simulink model "EV_TMS_MODEL"  (R2024a)
settings: Solver=VariableStepAuto  StartTime=0.0  StopTime=1000  RelTol=1e-3
values from neighbouring files (symbols this model uses):
  air_density = 1.225    [model_script.m]
  battery_C1_LUT = [1913.6 12447 30609 ... (first row only)    [model_script.m]
  battery_capacity_LUT = [280.081 276.25 276.392]    [model_script.m]
  battery_cell_cp = 795    [model_script.m]
  battery_cell_mass = 2.5    [model_script.m]
  battery_Em_LUT = [3.4966 3.5057 3.5148 ... (first row only)    [model_script.m]
  battery_N_cells = 20    [model_script.m]
  battery_Qe_init = 0    [model_script.m]
  battery_R0_LUT = [0.0117 0.0085 0.009 ... (first row only)    [model_script.m]
  battery_R1_LUT = [0.0109 0.0029 0.0013 ... (first row only)    [model_script.m]
  battery_SOC_LUT = [0; 0.1; 0.25; 0.5; 0.75; 0.9; 1]    [model_script.m]
  battery_T_init = -10    [model_script.m]
  battery_temperature_LUT = [-10 0 5 20 40]    [model_script.m]
  cabin_doors_conductivity = 0.2    [model_script.m]
  cabin_glass_conductivity = 1    [model_script.m]
  cabin_roof_conductivity = 0.2    [model_script.m]
  cabin_T_init = -10    [model_script.m]
  coolant_channel_D = 0.0092    [model_script.m]
  coolant_pipe_D = 0.02    [model_script.m]
  coolant_T_init = 30    [model_script.m]
  coolant_tank_volume = 5    [model_script.m]
  CoolingPower_kW = 3    [model_script.m]
  duct_W = 0.2    [model_script.m]
  evap_superheat_temp = 5    [model_script.m]
  pump_speed_max = 3000    [model_script.m]
  refrigerant_massflowrate = CoolingPower_kW/(evap_outlet_enthalpy-evap_inlet_enthalpy)    (= 0.0184049079755)    [model_script.m]
  RPM_Compressor_nominal = 1000    [model_script.m]
  RPM_CondFan = 3000    [model_script.m]
  RPM_EvapFan = 3000    [model_script.m]
  T_set = 20    [model_script.m]
  tube_D = 0.01    [model_script.m]
  VolFlowrate_CondenserFan = condenser_air_massflowrate/air_density    (= 0.408163265306)    [model_script.m]
  VolFlowRate_CoolantRadiatorFan = 0.5    [model_script.m]
  VolFlowRate_EvapFan = evap_air_massflowrate/air_density    (= 0.487359122754)    [model_script.m]
undefined symbols (not defined in the file or in its folder): bulb, inlet
libraries: fl_lib x238, nesl_utility x75, SimscapeFluids_lib x25, LiBatteryElements_lib x16, simulink_extras x9, slpidlib x3, autolibshared x1, SignalEditorBlockLib x1
(part 1 of 7)
settings Model: Creator=sairathik  LastModifiedBy=sairathik
settings DataIOCC: LoggingToFile=on
settings SimscapeCC: SimscapeLogType=all

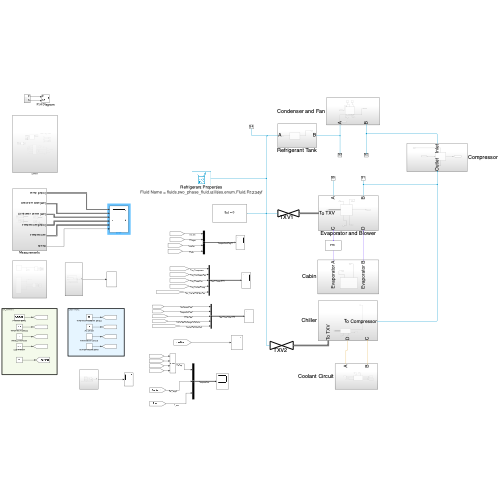
[thumbnail: Simulink's stored preview of the top-level diagram]
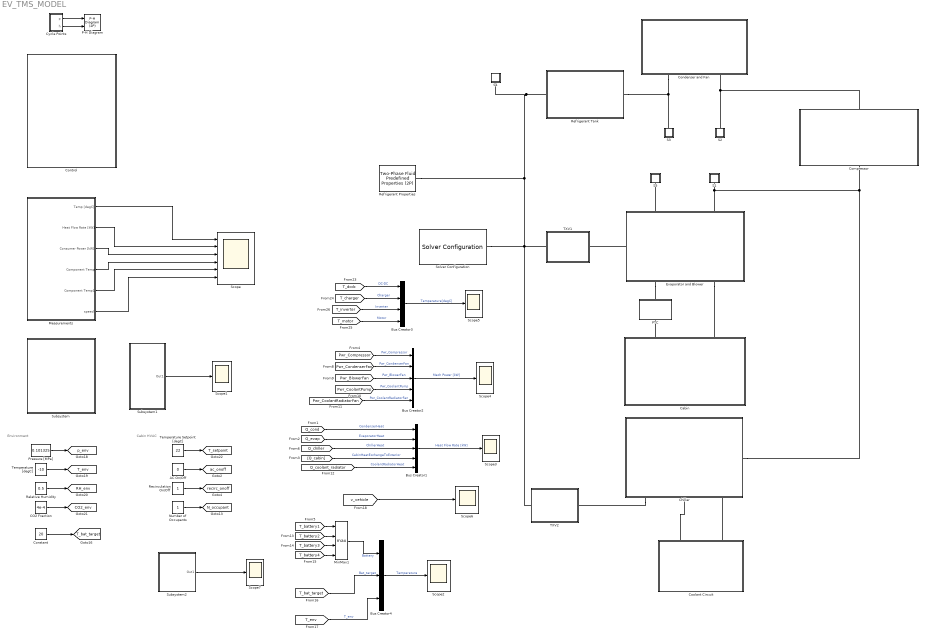
== system EV_TMS_MODEL ==
  note: Cabin HVAC
  note: Environment
  AC On/Off : Constant  Value=0
  Bus Creator1 : BusCreator  Inputs=5
  Bus Creator2 : BusCreator  Inputs=5
  Bus Creator3 : BusCreator  Inputs=4
  Bus Creator4 : BusCreator  Inputs=3
  CO2 Fraction : Constant  Value=4e-4
  Cabin : Subsystem
  Chiller : Subsystem
      settings: PortSchema="{\"entries\":[{\"content\":{\"sides\":[{\"content\":{\"connectorIds\":[\"LConn1\",\"LConn2\",\"LConn3\"]},\"type\":\"ConnectorPlacement.EquallySpacedRectSide\",\"uuid\":\"34bef901-d7f5-4aae-8cd5-5259b1e8621f\"},{\"content\":{\"side\":\"RIGHT\"},\"type\":\"ConnectorPlacement.EquallySpacedRectSide\",\"uuid\":\"b01a48cc-07de-4dff-b61c-731d99d876f5\"},{\"content\":{\"side\":\"TOP\"},\"type\":\"ConnectorPlacement.EquallySpacedRectSide\",\"uuid\":\"208c4f13-23a8-48df-b330-7ce2967b477c\"},{\"content\":{\"connectorIds\":[\"RConn1\"],\"side\":\"BOTTOM\"},\"type\":\"ConnectorPlacement.EquallySpacedRectSide\",\"uuid\":\"3f2d2c72-c43a-4e73-a9fe-b270fdc2a992\"}]},\"type\":\"ConnectorPlacement.EquallySpacedConnector\",\"uuid\":\"b9cc5a63-1194-4be5-9345-4e1b905bf50a\"}],\"packageUris\":[\"http://schema.mathworks.com/mf0/Connector/R2020b\"],\"version\":\"1.0\"}"
  Compressor : Subsystem
  Condenser and Fan : Subsystem
  Constant : Constant  Value=20
  Control : Subsystem
  Coolant Circuit : Subsystem
  Cycle Points : Subsystem
  Evaporator and Blower : Subsystem
      settings: PortSchema="{\"entries\":[{\"content\":{\"sides\":[{\"content\":{\"connectorIds\":[\"LConn1\"]},\"type\":\"ConnectorPlacement.EquallySpacedRectSide\",\"uuid\":\"157f3fa2-0ecb-424c-8810-23d73986b741\"},{\"content\":{\"side\":\"RIGHT\"},\"type\":\"ConnectorPlacement.EquallySpacedRectSide\",\"uuid\":\"a4531bf6-8393-4021-8b08-3c66bf47a331\"},{\"content\":{\"connectorIds\":[\"LConn2\",\"LConn3\"],\"side\":\"TOP\"},\"type\":\"ConnectorPlacement.EquallySpacedRectSide\",\"uuid\":\"3b910221-5f3a-43b2-b1cc-6f755753cce0\"},{\"content\":{\"connectorIds\":[\"RConn1\",\"RConn2\"],\"side\":\"BOTTOM\"},\"type\":\"ConnectorPlacement.EquallySpacedRectSide\",\"uuid\":\"a4f12d0e-e514-4dfe-871d-1a4bb02b790e\"}]},\"type\":\"ConnectorPlacement.EquallySpacedConnector\",\"uuid\":\"e79167fd-0289-46ca-9807-ec7889629a3a\"}],\"packageUris\":[\"http://schema.mathworks.com/mf0/Connector/R2020b\"],\"version\":\"1.0\"}"
  Measurements : Subsystem
  MinMax1 : MinMax  Function=max  Inputs=4
  Number of Occupants : Constant
  P-H Diagram : SimscapeFluids_lib/Two-Phase Fluid/Utilities/P-H Diagram (2P)
  PTC : Subsystem  Tag=PublishSubsystem
      mask Display: disp(get_param(gcb, 'Name'))
  Pressure [MPa] : Constant  Value=0.101325
  Recirculation On/Off : Constant
  Refrigerant Properties : SimscapeFluids_lib/Two-Phase Fluid/Utilities/Two-Phase Fluid Predefined Properties (2P)  fluid=fluids.two_phase_fluid.utilities.enum.Fluid.R1234yf  p_atm=0.6102 MPa  properties_range_check=simscape.enum.assert.action.error  q_rev=0.01 Pa
      settings: AttributesFormatString=Fluid Name = %<fluid>
  Refrigerant Tank : Subsystem
  Relative Humidity : Constant  Value=0.5
  S1 : Subsystem
      mask Display: disp(get_param(gcb, 'Name'))
  S2 : Subsystem
      mask Display: disp(get_param(gcb, 'Name'))
  S3 : Subsystem
      settings: PortSchema="{\"entries\":[{\"content\":{\"sides\":[{\"content\":{\"connectorIds\":[]},\"type\":\"ConnectorPlacement.EquallySpacedRectSide\",\"uuid\":\"16f002de-4636-401c-8be6-20698decbc91\"},{\"content\":{\"connectorIds\":[],\"side\":\"RIGHT\"},\"type\":\"ConnectorPlacement.EquallySpacedRectSide\",\"uuid\":\"76477188-11a3-4efa-a92e-0d269d480ac3\"},{\"content\":{\"connectorIds\":[],\"side\":\"TOP\"},\"type\":\"ConnectorPlacement.EquallySpacedRectSide\",\"uuid\":\"05fe64e4-9858-4712-a671-6ec27cab8615\"},{\"content\":{\"connectorIds\":[\"RConn1\"],\"side\":\"BOTTOM\"},\"type\":\"ConnectorPlacement.EquallySpacedRectSide\",\"uuid\":\"ddad7bbe-c900-450c-9863-e8fdc2274286\"}]},\"type\":\"ConnectorPlacement.EquallySpacedConnector\",\"uuid\":\"12bdef6d-66b8-4c10-9167-065994fcb3b8\"}],\"packageUris\":[\"http://schema.mathworks.com/mf0/Connector/R2020b\"],\"version\":\"1.0\"}"
      mask Display: disp(get_param(gcb, 'Name'))
  S4 : Subsystem
      mask Display: disp(get_param(gcb, 'Name'))
  S5 : Subsystem
      mask Display: disp(get_param(gcb, 'Name'))
  Scope : Scope  NumInputPorts=6
  Scope{1..7} (7 alike) : Scope
  Solver Configuration : nesl_utility/Solver Configuration  PhysicalDomain=network_engine_domain  SubClassName=solver  LeftPortType=input  RightPortType=generic  Tones=[]  Harmonics=[]  SimulateNoise=off  Profile=off  UseLocalSampling=off  EnableSwitchedLinearOptims=on  FrequencyDomain=off  UseCCode=off  RelTol=0.001  AbsTol=0.001  MinStep=1e-09  ToWorkspace=off  RevertToSquareIcSolve=off  NumHomotopyIterations=100  PhasorMode=off  PhasorModeNumHarmonics=1  ConsistencySolver=NEWTON_XTOL_AFTER_FTOL  IndexReductionMethod=DerivativeReplacement  DoDC=off  ResidualTolerance=1e-6  ConsistencyTolSource=GLOBAL  ConsistencyAbsTol=0.001  ConsistencyRelTol=0.001  ConsistencyTolFactor=0.001  UseLocalSolver=off  LocalSolverChoice=NE_BACKWARD_EULER_ADVANCER  ResolveIndetEquations=on  FunctionEvalNumThread=1  LocalSolverSampleTime=0.01  DoFixedCost=off  MaxNonlinIter=100  MaxModeIter=10  ComputeImpulses=off  ImpulseIterations=2  LinearAlgebra=auto  LinearAlgebraNumThread=0  EquationFormulation=NE_TIME_EF  DelaysMemoryBudget=1024  AutomaticFiltering=on  FilteringTimeConstant=0.001  PartitionStorageMethod=AS_NEEDED  PartitionMemoryBudget=1024  PartitionMethod=ROBUST  MultibodyUseLocalSolver=off  MultibodyLocalSolverChoice=ODE1  MultibodyLocalSolverSampleTime=0.001
  Subsystem : Subsystem
  Subsystem1 : Subsystem
  Subsystem2 : Subsystem
  TXV1 : Subsystem  Tag=PublishSubsystem
      mask Display:
      | color('white')
      | plot(100, 100)
      | plot(-100, -100)
      | color('black')
      | 
      | plot([0 -100 -100 0], [0 50 -50 0])
      | plot([0 100 100 0], [0 50 -50 0])
      | 
      | text(-50,60,get_param(gcb, 'Name'))
  TXV2 : Subsystem  Tag=PublishSubsystem
      mask Display:
      | color('white')
      | plot(100, 100)
      | plot(-100, -100)
      | color('black')
      | 
      | plot([0 -100 -100 0], [0 50 -50 0])
      | plot([0 100 100 0], [0 50 -50 0])
      | 
      | text(-50,60,get_param(gcb, 'Name'))
  Temperature Setpoint [degC] : Constant  Value=22
  Temperature [degC] : Constant  Value=-10
  tag scope: CO2_env=global, N_occupant=global, RH_env=global, T_bat_target=global, T_env=global, T_setpoint=global, ac_onoff=global, p_env=global, recirc_onoff=global
  wires:
  Cycle Points/2(h) -> P-H Diagram/2
  Cycle Points/1(p) -> P-H Diagram/1
  AC On/Off/1 -> [ac_onoff]
  Pressure [MPa]/1 -> [p_env]
  CO2 Fraction/1 -> [CO2_env]
  Number of Occupants/1 -> [N_occupant]
  Relative Humidity/1 -> [RH_env]
  Temperature Setpoint [degC]/1 -> [T_setpoint]
  Recirculation On/Off/1 -> [recirc_onoff]
  Temperature [degC]/1 -> [T_env]
  Measurements/1(Temp [degC]) -> Scope/1
  Measurements/2(Heat Flow Rate [kW]) -> Scope/2
  Measurements/3(Consumer Power [kW]) -> Scope/3
  Measurements/4(Component Temp) -> Scope/4
  Constant/1 -> [T_bat_target]
  Measurements/5(Component Temp1) -> Scope/5
  Subsystem1/1(Out1) -> Scope1/1
  Bus Creator4/1 -> Scope2/1  "Temperature"
  MinMax1/1 -> Bus Creator4/1  "Battery"
  [T_battery1] -> MinMax1/1
  [T_battery3] -> MinMax1/3
  [T_battery2] -> MinMax1/2
  [T_env] -> Bus Creator4/3  "T_env"
  [T_bat_target] -> Bus Creator4/2  "Bat_target"
  [T_battery4] -> MinMax1/4
  [Q_cond] -> Bus Creator1/1  "CondenserHeat"
  [Q_evap] -> Bus Creator1/2  "EvaporatorHeat"
  [Q_chiller] -> Bus Creator1/3  "ChillerHeat"
  [Q_cabin] -> Bus Creator1/4  "CabinHeatExchangeToExterior"
  [Q_coolant_radiator] -> Bus Creator1/5  "CoolantRadiatorHeat"
  Bus Creator1/1 -> Scope3/1  "Heat Flow Rate [kW]"
  [Pwr_CoolantPump] -> Bus Creator2/4  "Pwr_CoolantPump"
  [Pwr_CoolantRadiatorFan] -> Bus Creator2/5  "Pwr_CoolantRadiatorFan"
  [Pwr_CondenserFan] -> Bus Creator2/2  "Pwr_CondenserFan"
  Bus Creator2/1 -> Scope4/1  "Mech Power [kW]"
  [Pwr_Compressor] -> Bus Creator2/1  "Pwr_Compressor"
  [Pwr_BlowerFan] -> Bus Creator2/3  "Pwr_BlowerFan"
  Bus Creator3/1 -> Scope5/1  "Temperature[degC]"
  [T_charger] -> Bus Creator3/2  "Charger"
  [T_dcdc] -> Bus Creator3/1  "DC-DC"
  [T_motor] -> Bus Creator3/4  "Motor"
  [T_inverter] -> Bus Creator3/3  "Inverter"
  Measurements/6(speed) -> Scope/6
  [v_vehicle] -> Scope6/1
  Subsystem2/1(Out1) -> Scope7/1
  connections:
  S1/LConn1 -- Chiller/RConn1 -- Compressor/LConn1 -- Evaporator and Blower/LConn3
  Solver Configuration/RConn1 -- TXV2/RConn1 -- Refrigerant Properties/RConn1 -- Refrigerant Tank/LConn1 -- S4/LConn1 -- TXV1/RConn1
  S2/LConn1 -- Compressor/RConn1 -- Condenser and Fan/RConn2
  Condenser and Fan/RConn1 -- Refrigerant Tank/RConn1 -- S3/RConn1
  S5/LConn1 -- Evaporator and Blower/LConn2
  Evaporator and Blower/LConn1 -- TXV1/LConn1
  Evaporator and Blower/RConn1 -- PTC/RConn1
  PTC/LConn1 -- Cabin/LConn1
  Evaporator and Blower/RConn2 -- Cabin/LConn2
  Chiller/LConn1 -- TXV2/LConn1
  Coolant Circuit/LConn1 -- Chiller/LConn2
  Coolant Circuit/LConn2 -- Chiller/LConn3

== system EV_TMS_MODEL/Cabin ==
  Cabin : Subsystem
      settings: PortSchema="{\"entries\":[{\"content\":{\"sides\":[{\"content\":{},\"type\":\"ConnectorPlacement.EquallySpacedRectSide\",\"uuid\":\"5cf57e4f-975f-4b0b-a8e8-bf86758a11fa\"},{\"content\":{\"side\":\"RIGHT\"},\"type\":\"ConnectorPlacement.EquallySpacedRectSide\",\"uuid\":\"7f477a27-3a34-4ed6-85c3-331630c97133\"},{\"content\":{\"connectorIds\":[\"LConn1\",\"LConn2\"],\"side\":\"TOP\"},\"type\":\"ConnectorPlacement.EquallySpacedRectSide\",\"uuid\":\"743b5c17-84cf-4a2e-818e-c1a69eb195e5\"}]},\"type\":\"ConnectorPlacement.EquallySpacedConnector\",\"uuid\":\"4a6d6dd0-79df-4460-8879-70a258476fa5\"}],\"packageUris\":[\"http://schema.mathworks.com/mf0/Connector/R2020b\"],\"version\":\"1.0\"}"
      mask Display: disp(get_param(gcb, 'Name'));
  Evaporator A : PMIOPort  Side=Left
  Evaporator B : PMIOPort  Port=2  Side=Left
  connections:
  Evaporator B/RConn1 -- Cabin/LConn2
  Evaporator A/RConn1 -- Cabin/LConn1

== system EV_TMS_MODEL/Chiller ==
  Chiller : Subsystem  Tag=PublishSubsystem
      settings: PortSchema="{\"entries\":[{\"content\":{\"sides\":[{\"content\":{\"connectorIds\":[\"Out1\",\"LConn1\"]},\"type\":\"ConnectorPlacement.EquallySpacedRectSide\",\"uuid\":\"684495fe-43ac-42d2-91f9-c1083f68d635\"},{\"content\":{\"connectorIds\":[\"RConn1\"],\"side\":\"RIGHT\"},\"type\":\"ConnectorPlacement.EquallySpacedRectSide\",\"uuid\":\"acb3d27a-41e1-4bfe-a4d6-36d5666e4ba3\"},{\"content\":{\"connectorIds\":[\"LConn2\",\"LConn3\"],\"side\":\"TOP\"},\"type\":\"ConnectorPlacement.EquallySpacedRectSide\",\"uuid\":\"cdadeb40-472c-4edb-91b8-a2216ea85c99\"},{\"content\":{\"side\":\"BOTTOM\"},\"type\":\"ConnectorPlacement.EquallySpacedRectSide\",\"uuid\":\"46a4312c-e637-44ea-bfb3-e887da9d9904\"}]},\"type\":\"ConnectorPlacement.EquallySpacedConnector\",\"uuid\":\"20e25167-e167-414a-8c66-12b35ae5ef5e\"}],\"packageUris\":[\"http://schema.mathworks.com/mf0/Connector/R2020b\"],\"version\":\"1.0\"}"
      mask Display: disp(get_param(gcb, 'Name'));
  To TXV : PMIOPort  Side=Left
  D : PMIOPort  Port=2  Side=Left
  C : PMIOPort  Port=3  Side=Left
  To Compressor : PMIOPort  Port=4  Side=Right
  tag scope: Q_chiller=global
  wires:
  Chiller/1(Heat flow rate [kW]) -> [Q_chiller]  "Q_chiller"
  connections:
  C/RConn1 -- Chiller/LConn2
  Chiller/LConn1 -- To Compressor/RConn1
  D/RConn1 -- Chiller/LConn3
  Chiller/RConn1 -- To TXV/RConn1

== system EV_TMS_MODEL/Compressor ==
  Compressor : Subsystem
      settings: PortSchema="{\"entries\":[{\"content\":{\"sides\":[{\"content\":{\"connectorIds\":[\"LConn1\"]},\"type\":\"ConnectorPlacement.EquallySpacedRectSide\",\"uuid\":\"87497da4-7fcd-4c39-9d14-dd80365934db\"},{\"content\":{\"connectorIds\":[\"RConn1\"],\"side\":\"RIGHT\"},\"type\":\"ConnectorPlacement.EquallySpacedRectSide\",\"uuid\":\"c29b3d2b-7130-4a2f-8dcb-58b301edb84d\"},{\"content\":{\"connectorIds\":[\"In1\"],\"side\":\"TOP\"},\"type\":\"ConnectorPlacement.EquallySpacedRectSide\",\"uuid\":\"6b0e1579-3829-4056-a1f0-26424a36bca1\"},{\"content\":{\"connectorIds\":[\"Out1\"],\"side\":\"BOTTOM\"},\"type\":\"ConnectorPlacement.EquallySpacedRectSide\",\"uuid\":\"6b49380d-e724-4e3a-86e0-6bc21724e354\"}]},\"type\":\"ConnectorPlacement.EquallySpacedConnector\",\"uuid\":\"16d6c8a7-8265-44ec-91d1-631bbb83e0af\"}],\"packageUris\":[\"http://schema.mathworks.com/mf0/Connector/R2020b\"],\"version\":\"1.0\"}"
      mask Display: disp(get_param(gcb, 'Name'));
  Inlet : PMIOPort  Side=Right
  Outlet : PMIOPort  Port=2  Side=Left
  tag scope: Pwr_Compressor=global
  wires:
  [compressor] -> Compressor/1(Compressor On/Off)
  Compressor/1(Power [kW]) -> [Pwr_Compressor]  "Pwr_Compressor"
  connections:
  Compressor/LConn1 -- Outlet/RConn1
  Compressor/RConn1 -- Inlet/RConn1

== system EV_TMS_MODEL/Condenser and Fan ==
  Air In : fl_lib/Moist Air/Elements/Reservoir (MA)  pressure_spec=foundation.enum.pressure_spec.specified  reservoir_pressure=0.101325 MPa  temperature_spec=foundation.enum.temperature_spec.specified  reservoir_temperature=T_env degC  moisture_spec=foundation.enum.moisture_spec.relative_humidity  reservoir_RH=0.5  reservoir_x_w=0.01  reservoir_y_w=0.01  reservoir_HR=0.01  reservoir_Tw=287 K  trace_gas_spec=foundation.enum.trace_gas_spec.mole_fraction  reservoir_x_g=0.001  reservoir_y_g=0  RH_ws=1  area_A=duct_W^2 m^2
      settings: AttributesFormatString=temperature= %<reservoir_temperature>
  Air Out : fl_lib/Moist Air/Elements/Reservoir (MA)  pressure_spec=foundation.enum.pressure_spec.specified  reservoir_pressure=0.101325 MPa  temperature_spec=foundation.enum.temperature_spec.specified  reservoir_temperature=T_env degC  moisture_spec=foundation.enum.moisture_spec.relative_humidity  reservoir_RH=0.5  reservoir_x_w=0.01  reservoir_y_w=0.01  reservoir_HR=0.01  reservoir_Tw=287 K  trace_gas_spec=foundation.enum.trace_gas_spec.mole_fraction  reservoir_x_g=0.001  reservoir_y_g=0  RH_ws=1  area_A=duct_W^2 m^2
      settings: AttributesFormatString=temperature= %<reservoir_temperature>
  Condenser and Fan : Subsystem
      mask Display: disp(get_param(gcb, 'Name'));
  A : PMIOPort  Side=Right
  B : PMIOPort  Port=2  Side=Right
  tag scope: Pwr_CondenserFan=global, Q_cond=global
  wires:
  Condenser and Fan/2(Fan Power [kW]) -> [Q_cond]  "Q_condenser"
  Condenser and Fan/1(Heat Power [kW]) -> [Pwr_CondenserFan]  "Pwr_CondenserFan"
  [condenser_fan] -> Condenser and Fan/1(Fan On/Off)
  connections:
  Air Out/LConn1 -- Condenser and Fan/LConn2
  Condenser and Fan/LConn1 -- Air In/LConn1
  B/RConn1 -- Condenser and Fan/RConn2
  A/RConn1 -- Condenser and Fan/RConn1

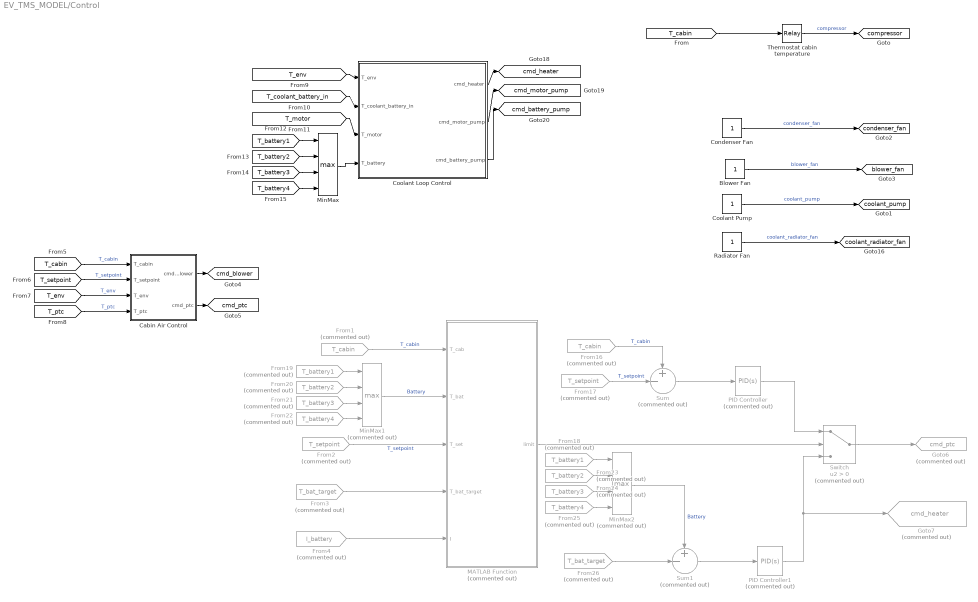
== system EV_TMS_MODEL/Control ==
  Blower Fan : Constant  SampleTime=1
  Cabin Air Control : Subsystem
  Condenser Fan : Constant  SampleTime=1
  Coolant Loop Control : Subsystem
  Coolant Pump : Constant  SampleTime=1
  From1 : From  Commented=on  GotoTag=T_cabin  TagVisibility=global
  From16 : From  Commented=on  GotoTag=T_cabin  TagVisibility=global
  From17 : From  Commented=on  GotoTag=T_setpoint  TagVisibility=global
  From18 : From  Commented=on  GotoTag=T_battery1  TagVisibility=global
  From19 : From  Commented=on  GotoTag=T_battery1  TagVisibility=global
  From2 : From  Commented=on  GotoTag=T_setpoint  TagVisibility=global
  From20 : From  Commented=on  GotoTag=T_battery2  TagVisibility=global
  From21 : From  Commented=on  GotoTag=T_battery3  TagVisibility=global
  From22 : From  Commented=on  GotoTag=T_battery4  TagVisibility=global
  From23 : From  Commented=on  GotoTag=T_battery2  TagVisibility=global
  From24 : From  Commented=on  GotoTag=T_battery3  TagVisibility=global
  From25 : From  Commented=on  GotoTag=T_battery4  TagVisibility=global
  From26 : From  Commented=on  GotoTag=T_bat_target  TagVisibility=global
  From3 : From  Commented=on  GotoTag=T_bat_target  TagVisibility=global
  From4 : From  Commented=on  GotoTag=I_battery  TagVisibility=global
  Goto6 : Goto  Commented=on  GotoTag=cmd_ptc  TagVisibility=global
  Goto7 : Goto  Commented=on  GotoTag=cmd_heater  TagVisibility=global
  MATLAB Function : MATLAB Function  Commented=on  TreatAsAtomicUnit=on
  MinMax : MinMax  Function=max  Inputs=4
  MinMax1 : MinMax  Commented=on  Function=max  Inputs=4
  MinMax2 : MinMax  Commented=on  Function=max  Inputs=4
  PID Controller : slpidlib/PID Controller  Commented=on  Controller=PID  Form=Parallel  TimeDomain=Continuous-time  UseExternalTs=off  SampleTime=-1  IntegratorMethod=Forward Euler  FilterMethod=Forward Euler  ControllerParametersSource=internal  P=1  I=1  UseKiTs=off  D=0  UseExternalDerivativeSource=off  N=100  UseFilter=on  TunerSelectOption=Transfer Function Based (PID Tuner App)  InitialConditionSource=internal  InitialConditionForIntegrator=0  InitialConditionForFilter=0  DifferentiatorICPrevScaledInput=0  ExternalReset=none  TrackingMode=off  Kt=1  LimitOutput=off  SatLimitsSource=internal  UpperSaturationLimit=inf  LowerSaturationLimit=-inf  LinearizeAsGain=on  AntiWindupMode=none  Kb=1  LimitIntegrator=off  UpperIntegratorSaturationLimit=inf  LowerIntegratorSaturationLimit=-inf  POutMin=[]  POutMax=[]  IOutMin=[]  IOutMax=[]  DOutMin=[]  DOutMax=[]  NOutMin=[]  NOutMax=[]  SumOutMin=[]  SumOutMax=[]  SaturationOutMin=[]  SaturationOutMax=[]  PParamMin=[]  PParamMax=[]  IParamMin=[]  IParamMax=[]  DParamMin=[]  DParamMax=[]  NParamMin=[]  NParamMax=[]  KbParamMin=[]  KbParamMax=[]  KtParamMin=[]  KtParamMax=[]  KbOutMin=[]  KbOutMax=[]  KtOutMin=[]  KtOutMax=[]  IntegratorOutMin=[]  IntegratorOutMax=[]  FilterOutMin=[]  FilterOutMax=[]  SumI1OutMin=[]  SumI1OutMax=[]  SumI2OutMin=[]  SumI2OutMax=[]  SumI3OutMin=[]  SumI3OutMax=[]  SumI4OutMin=[]  SumI4OutMax=[]  SumDOutMin=[]  SumDOutMax=[]  DifferentiatorOutMin=[]  DifferentiatorOutMax=[]  FilterDiffOutCoefMin=[]  FilterDiffOutCoefMax=[]  ReciprocalOutMin=[]  ReciprocalOutMax=[]  SumDenOutMin=[]  SumDenOutMax=[]  SumNumOutMin=[]  SumNumOutMax=[]  DivideOutMin=[]  DivideOutMax=[]  UdiffTsProdOutMin=[]  UdiffTsProdOutMax=[]  NTsProdOutMin=[]  NTsProdOutMax=[]  UintegralTsProdOutMin=[]  UintegralTsProdOutMax=[]  UngainTsProdOutMin=[]  UngainTsProdOutMax=[]  ClampingZeroOutDataTypeStr=Inherit: Inherit via back propagation  ClampingZeroOutMin=[]  ClampingZeroOutMax=[]  FilterDenConstantOutDataTypeStr=Inherit: Inherit via back propagation  FilterDenConstantOutMin=[]  FilterDenConstantOutMax=[]  PCopyOutDataTypeStr=Inherit: Inherit via back propagation  PCopyOutMin=[]  PCopyOutMax=[]  NCopyOutDataTypeStr=Inherit: Inherit via back propagation  NCopyOutMin=[]  NCopyOutMax=[]  IntegratorContinuousStateAttributes=''  IntegratorStateMustResolveToSignalObject=off  IntegratorRTWStateStorageClass=Auto  FilterContinuousStateAttributes=''  FilterStateMustResolveToSignalObject=off  FilterRTWStateStorageClass=Auto  ParallelPVariant=InternalParameters  IdealPVariant=Disabled  IVariant=InternalParameters  DVariant=InternalParameters  IntegratorVariant=Continuous  SatVariant=Disabled  AWVariant=Passthrough  PCopyVariant=Disabled  TRVariant=Disabled  FdbkBlocksVariant=Forward  IdealPFdbkVariant=Disabled  SatFdbkVariant=Disabled  DerivativeFilterVariant=ContFilter  NVariant=InternalParameters  NCopyVariant=Disabled  FilterICVariant=InternalICsFilter  IntegratorICVariant=InternalICs  ExternalResetVariant=Disabled  TRSumVariant=Passthrough  SumFdbkVariant=Disabled  SumVariant=Sum_PID  TsampFilterVariant=InternalTs  TsampNgainVariant=Passthrough  TsampIntegralVariant=Disabled_SignalSpec  ExternalSaturationOutDataTypeStr=Inherit: Same as second input  DerivativeSourceVariant=ErrorSignal
  PID Controller1 : slpidlib/PID Controller  Commented=on  Controller=PID  Form=Parallel  TimeDomain=Continuous-time  UseExternalTs=off  SampleTime=-1  IntegratorMethod=Forward Euler  FilterMethod=Forward Euler  ControllerParametersSource=internal  P=1  I=1  UseKiTs=off  D=0.1  UseExternalDerivativeSource=off  N=100  UseFilter=on  TunerSelectOption=Transfer Function Based (PID Tuner App)  InitialConditionSource=internal  InitialConditionForIntegrator=0  InitialConditionForFilter=0  DifferentiatorICPrevScaledInput=0  ExternalReset=none  TrackingMode=off  Kt=1  LimitOutput=off  SatLimitsSource=internal  UpperSaturationLimit=inf  LowerSaturationLimit=-inf  LinearizeAsGain=on  AntiWindupMode=none  Kb=1  LimitIntegrator=off  UpperIntegratorSaturationLimit=inf  LowerIntegratorSaturationLimit=-inf  POutMin=[]  POutMax=[]  IOutMin=[]  IOutMax=[]  DOutMin=[]  DOutMax=[]  NOutMin=[]  NOutMax=[]  SumOutMin=[]  SumOutMax=[]  SaturationOutMin=[]  SaturationOutMax=[]  PParamMin=[]  PParamMax=[]  IParamMin=[]  IParamMax=[]  DParamMin=[]  DParamMax=[]  NParamMin=[]  NParamMax=[]  KbParamMin=[]  KbParamMax=[]  KtParamMin=[]  KtParamMax=[]  KbOutMin=[]  KbOutMax=[]  KtOutMin=[]  KtOutMax=[]  IntegratorOutMin=[]  IntegratorOutMax=[]  FilterOutMin=[]  FilterOutMax=[]  SumI1OutMin=[]  SumI1OutMax=[]  SumI2OutMin=[]  SumI2OutMax=[]  SumI3OutMin=[]  SumI3OutMax=[]  SumI4OutMin=[]  SumI4OutMax=[]  SumDOutMin=[]  SumDOutMax=[]  DifferentiatorOutMin=[]  DifferentiatorOutMax=[]  FilterDiffOutCoefMin=[]  FilterDiffOutCoefMax=[]  ReciprocalOutMin=[]  ReciprocalOutMax=[]  SumDenOutMin=[]  SumDenOutMax=[]  SumNumOutMin=[]  SumNumOutMax=[]  DivideOutMin=[]  DivideOutMax=[]  UdiffTsProdOutMin=[]  UdiffTsProdOutMax=[]  NTsProdOutMin=[]  NTsProdOutMax=[]  UintegralTsProdOutMin=[]  UintegralTsProdOutMax=[]  UngainTsProdOutMin=[]  UngainTsProdOutMax=[]  ClampingZeroOutDataTypeStr=Inherit: Inherit via back propagation  ClampingZeroOutMin=[]  ClampingZeroOutMax=[]  FilterDenConstantOutDataTypeStr=Inherit: Inherit via back propagation  FilterDenConstantOutMin=[]  FilterDenConstantOutMax=[]  PCopyOutDataTypeStr=Inherit: Inherit via back propagation  PCopyOutMin=[]  PCopyOutMax=[]  NCopyOutDataTypeStr=Inherit: Inherit via back propagation  NCopyOutMin=[]  NCopyOutMax=[]  IntegratorContinuousStateAttributes=''  IntegratorStateMustResolveToSignalObject=off  IntegratorRTWStateStorageClass=Auto  FilterContinuousStateAttributes=''  FilterStateMustResolveToSignalObject=off  FilterRTWStateStorageClass=Auto  ParallelPVariant=InternalParameters  IdealPVariant=Disabled  IVariant=InternalParameters  DVariant=InternalParameters  IntegratorVariant=Continuous  SatVariant=Disabled  AWVariant=Passthrough  PCopyVariant=Disabled  TRVariant=Disabled  FdbkBlocksVariant=Forward  IdealPFdbkVariant=Disabled  SatFdbkVariant=Disabled  DerivativeFilterVariant=ContFilter  NVariant=InternalParameters  NCopyVariant=Disabled  FilterICVariant=InternalICsFilter  IntegratorICVariant=InternalICs  ExternalResetVariant=Disabled  TRSumVariant=Passthrough  SumFdbkVariant=Disabled  SumVariant=Sum_PID  TsampFilterVariant=InternalTs  TsampNgainVariant=Passthrough  TsampIntegralVariant=Disabled_SignalSpec  ExternalSaturationOutDataTypeStr=Inherit: Same as second input  DerivativeSourceVariant=ErrorSignal
  Radiator Fan : Constant  SampleTime=1
  Sum : Sum  Commented=on  Inputs=+-|
  Sum1 : Sum  Commented=on  Inputs=+-|
  Switch : Switch  Commented=on  Criteria=u2 > Threshold  SaturateOnIntegerOverflow=off  InputSameDT=off
  Thermostat cabin temperature : Relay  OnSwitchValue=T_set + 1  OffSwitchValue=T_set  ZeroCross=off
  tag scope: blower_fan=global, cmd_battery_pump=global, cmd_blower=global, cmd_heater=global, cmd_motor_pump=global, cmd_ptc=global, compressor=global, condenser_fan=global, coolant_pump=global, coolant_radiator_fan=global
  wires:
  Thermostat cabin temperature/1 -> [compressor]  "compressor"
  [T_coolant_battery_in] -> Coolant Loop Control/2(T_coolant_battery_in)
  Coolant Loop Control/3(cmd_battery_pump) -> [cmd_battery_pump]
  [T_battery1] -> MinMax/1
  [T_battery4] -> MinMax/4
  [T_env] -> Coolant Loop Control/1(T_env)
  [T_cabin] -> Thermostat cabin temperature/1
  Coolant Loop Control/2(cmd_motor_pump) -> [cmd_motor_pump]
  [T_motor] -> Coolant Loop Control/3(T_motor)
  Radiator Fan/1 -> [coolant_radiator_fan]  "coolant_radiator_fan"
  [T_battery3] -> MinMax/3
  Coolant Pump/1 -> [coolant_pump]  "coolant_pump"
  [T_battery2] -> MinMax/2
  MinMax/1 -> Coolant Loop Control/4(T_battery)
  Condenser Fan/1 -> [condenser_fan]  "condenser_fan"
  Coolant Loop Control/1(cmd_heater) -> [cmd_heater]
  [T_env] -> Cabin Air Control/3(T_env)  "T_env"
  [T_cabin] -> Cabin Air Control/1(T_cabin)  "T_cabin"
  [T_setpoint] -> Cabin Air Control/2(T_setpoint)  "T_setpoint"
  Cabin Air Control/2(cmd_ptc) -> [cmd_ptc]
  [T_ptc] -> Cabin Air Control/4(T_ptc)  "T_ptc"
  Cabin Air Control/1(cmd_blower) -> [cmd_blower]
  From1/1 -> MATLAB Function/1(T_cab)  "T_cabin"
  From22/1 -> MinMax1/4
  From21/1 -> MinMax1/3
  From19/1 -> MinMax1/1
  MinMax1/1 -> MATLAB Function/2(T_bat)  "Battery"
  From20/1 -> MinMax1/2
  From2/1 -> MATLAB Function/3(T_set)  "T_setpoint"
  From3/1 -> MATLAB Function/4(T_bat_target)
  PID Controller/1 -> Switch/1
  MATLAB Function/1(limit) -> Switch/2
  PID Controller1/1 -> Switch/3, Goto7/1
  From4/1 -> MATLAB Function/5(I)
  Switch/1 -> Goto6/1
  From16/1 -> Sum/1  "T_cabin"
  From17/1 -> Sum/2  "T_setpoint"
  MinMax2/1 -> Sum1/1  "Battery"
  From25/1 -> MinMax2/4
  From18/1 -> MinMax2/1
  From24/1 -> MinMax2/3
  From23/1 -> MinMax2/2
  From26/1 -> Sum1/2
  Sum/1 -> PID Controller/1
  Sum1/1 -> PID Controller1/1
  Blower Fan/1 -> [blower_fan]  "blower_fan"

== system EV_TMS_MODEL/Coolant Circuit ==
  Coolant Circuit : Subsystem
      settings: PortSchema="{\"entries\":[{\"content\":{\"sides\":[{\"content\":{\"connectorIds\":[\"In1\",\"In2\",\"In3\"]},\"type\":\"ConnectorPlacement.EquallySpacedRectSide\",\"uuid\":\"61b3bd2b-efba-48b8-bc1e-7d5fd1f93ea8\"},{\"content\":{\"connectorIds\":[\"Out1\",\"Out2\",\"Out3\",\"Out4\"],\"side\":\"RIGHT\"},\"type\":\"ConnectorPlacement.EquallySpacedRectSide\",\"uuid\":\"116770ca-4665-4fbe-8ef7-14ad65bf6363\"},{\"content\":{\"connectorIds\":[\"LConn1\",\"LConn2\"],\"side\":\"TOP\"},\"type\":\"ConnectorPlacement.EquallySpacedRectSide\",\"uuid\":\"8588f2a2-4124-40f5-9c68-b1b3344e047c\"}]},\"type\":\"ConnectorPlacement.EquallySpacedConnector\",\"uuid\":\"af351b75-e118-4ad1-8604-555a25a7fec0\"}],\"packageUris\":[\"http://schema.mathworks.com/mf0/Connector/R2020b\"],\"version\":\"1.0\"}"
      mask Display: disp(get_param(gcb, 'Name'));
  Heat flow rate to coolant [kW] : Constant  Value=0.5  SampleTime=1
  A : PMIOPort  Side=Left
  B : PMIOPort  Port=2  Side=Left
  tag scope: Pwr_CoolantPump=global, Pwr_CoolantRadiatorFan=global, Q_coolant_radiator=global, T_coolant=global
  wires:
  Heat flow rate to coolant [kW]/1 -> Coolant Circuit/1(Heat flow rate [kW])  "heat_flow_to_coolant_kW"
  Coolant Circuit/4(Radiator Heat Rate [kW]) -> [Q_coolant_radiator]  "Q_coolant_radiator"
  [coolant_pump] -> Coolant Circuit/2(Coolant Pump On/Off)
  Coolant Circuit/2(Pump Power [kW]) -> [Pwr_CoolantPump]  "Pwr_CoolantPump"
  Coolant Circuit/3(Radiator Fan Pwr [kW]) -> [Pwr_CoolantRadiatorFan]  "Pwr_CoolantRadiatorFan"
  [coolant_radiator_fan] -> Coolant Circuit/3(Radiator Fan On/Off)
  Coolant Circuit/1(Temperature [degC]) -> [T_coolant]  "T_coolant"
  connections:
  Coolant Circuit/LConn1 -- A/RConn1
  Coolant Circuit/LConn2 -- B/RConn1

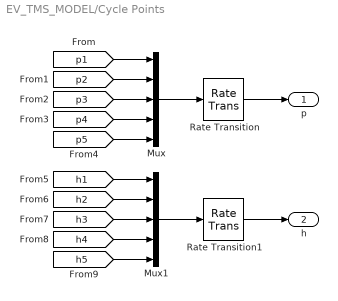
== system EV_TMS_MODEL/Cycle Points ==
  Mux : Mux  Inputs=5
  Mux1 : Mux  Inputs=5
  Rate Transition : RateTransition  OutPortSampleTime=10
  Rate Transition1 : RateTransition  OutPortSampleTime=10
  p : Outport
  h : Outport  Port=2
  wires:
  [p1] -> Mux/1
  [p2] -> Mux/2
  [p3] -> Mux/3
  [p4] -> Mux/4
  [p5] -> Mux/5
  Mux/1 -> Rate Transition/1
  Mux1/1 -> Rate Transition1/1
  [h5] -> Mux1/5
  [h4] -> Mux1/4
  [h3] -> Mux1/3
  [h2] -> Mux1/2
  [h1] -> Mux1/1
  Rate Transition/1 -> p/1
  Rate Transition1/1 -> h/1

== system EV_TMS_MODEL/Evaporator and Blower ==
  Evaporator and Blower Fan : Subsystem
      settings: PortSchema="{\"entries\":[{\"content\":{\"sides\":[{\"content\":{\"connectorIds\":[\"LConn1\",\"LConn2\"]},\"type\":\"ConnectorPlacement.EquallySpacedRectSide\",\"uuid\":\"94f743b0-016e-4f6c-ba37-cd5c9e5decb1\"},{\"content\":{\"connectorIds\":[\"RConn1\",\"RConn2\"],\"side\":\"RIGHT\"},\"type\":\"ConnectorPlacement.EquallySpacedRectSide\",\"uuid\":\"4e78d493-e8a5-489f-9c9b-6c9134237572\"},{\"content\":{\"connectorIds\":[\"LConn3\"],\"side\":\"TOP\"},\"type\":\"ConnectorPlacement.EquallySpacedRectSide\",\"uuid\":\"0b95dc75-9fe3-4b9e-8dc0-c99924a5b683\"},{\"content\":{\"connectorIds\":[\"Out1\"],\"side\":\"BOTTOM\"},\"type\":\"ConnectorPlacement.EquallySpacedRectSide\",\"uuid\":\"3125a7ac-4364-4843-9f9a-28cc842c280f\"}]},\"type\":\"ConnectorPlacement.EquallySpacedConnector\",\"uuid\":\"0b0f7158-6d74-402a-9204-25c9a3fd4099\"}],\"packageUris\":[\"http://schema.mathworks.com/mf0/Connector/R2020b\"],\"version\":\"1.0\"}"
      mask Display: disp(get_param(gcb, 'Name'));
  To TXV : PMIOPort  Side=Left
  A : PMIOPort  Port=2  Side=Left
  B : PMIOPort  Port=3  Side=Left
  C : PMIOPort  Port=4  Side=Right
  D : PMIOPort  Port=5  Side=Right
  tag scope: Q_evap=global
  wires:
  Evaporator and Blower Fan/1(Heat Power [kW]) -> [Q_evap]  "Q_evaporator"
  connections:
  B/RConn1 -- Evaporator and Blower Fan/LConn2
  Evaporator and Blower Fan/RConn1 -- C/RConn1
  Evaporator and Blower Fan/LConn3 -- To TXV/RConn1
  A/RConn1 -- Evaporator and Blower Fan/LConn1
  Evaporator and Blower Fan/RConn2 -- D/RConn1

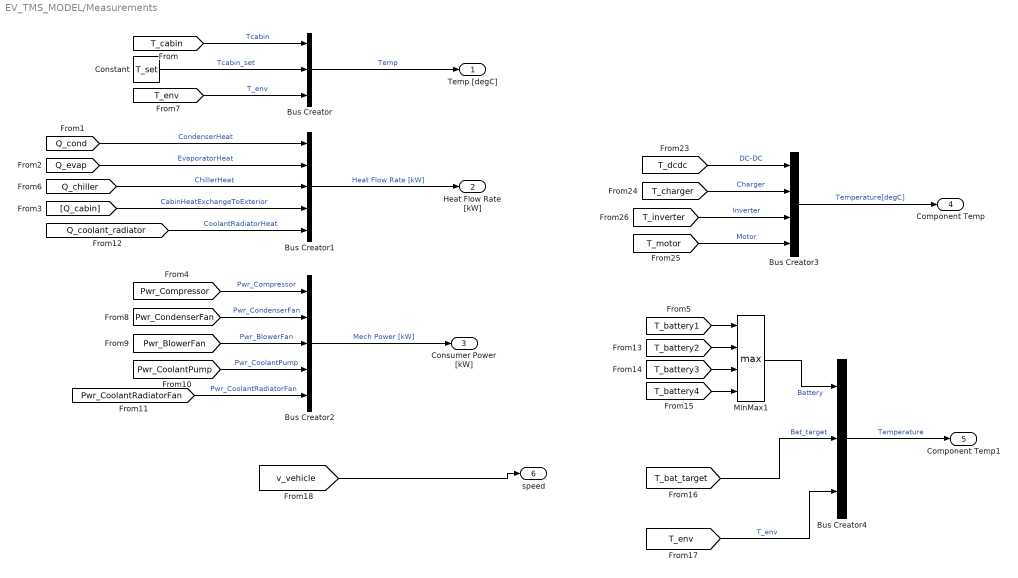
== system EV_TMS_MODEL/Measurements ==
  Bus Creator : BusCreator  Inputs=3
  Bus Creator1 : BusCreator  Inputs=5
  Bus Creator2 : BusCreator  Inputs=5
  Bus Creator3 : BusCreator  Inputs=4
  Bus Creator4 : BusCreator  Inputs=3
  Constant : Constant  Value=T_set
  MinMax1 : MinMax  Function=max  Inputs=4
  Temp [degC] : Outport
  Heat Flow Rate [kW] : Outport  Port=2
  Consumer Power [kW] : Outport  Port=3
  Component Temp : Outport  Port=4
  Component Temp1 : Outport  Port=5
  speed : Outport  Port=6
  wires:
  [T_cabin] -> Bus Creator/1  "Tcabin"
  Constant/1 -> Bus Creator/2  "Tcabin_set"
  Bus Creator/1 -> Temp [degC]/1  "Temp"
  Bus Creator1/1 -> Heat Flow Rate [kW]/1  "Heat Flow Rate [kW]"
  [Q_cond] -> Bus Creator1/1  "CondenserHeat"
  [Q_evap] -> Bus Creator1/2  "EvaporatorHeat"
  [Q_cabin] -> Bus Creator1/4  "CabinHeatExchangeToExterior"
  [Q_chiller] -> Bus Creator1/3  "ChillerHeat"
  [T_env] -> Bus Creator/3  "T_env"
  [Pwr_Compressor] -> Bus Creator2/1  "Pwr_Compressor"
  Bus Creator2/1 -> Consumer Power [kW]/1  "Mech Power [kW]"
  [Pwr_CondenserFan] -> Bus Creator2/2  "Pwr_CondenserFan"
  [Pwr_BlowerFan] -> Bus Creator2/3  "Pwr_BlowerFan"
  [Pwr_CoolantPump] -> Bus Creator2/4  "Pwr_CoolantPump"
  [Pwr_CoolantRadiatorFan] -> Bus Creator2/5  "Pwr_CoolantRadiatorFan"
  [Q_coolant_radiator] -> Bus Creator1/5  "CoolantRadiatorHeat"
  Bus Creator3/1 -> Component Temp/1  "Temperature[degC]"
  [T_dcdc] -> Bus Creator3/1  "DC-DC"
  [T_charger] -> Bus Creator3/2  "Charger"
  [T_motor] -> Bus Creator3/4  "Motor"
  [T_inverter] -> Bus Creator3/3  "Inverter"
  [T_battery4] -> MinMax1/4
  [T_battery3] -> MinMax1/3
  [T_battery1] -> MinMax1/1
  MinMax1/1 -> Bus Creator4/1  "Battery"
  [T_battery2] -> MinMax1/2
  [T_bat_target] -> Bus Creator4/2  "Bat_target"
  [T_env] -> Bus Creator4/3  "T_env"
  Bus Creator4/1 -> Component Temp1/1  "Temperature"
  [v_vehicle] -> speed/1

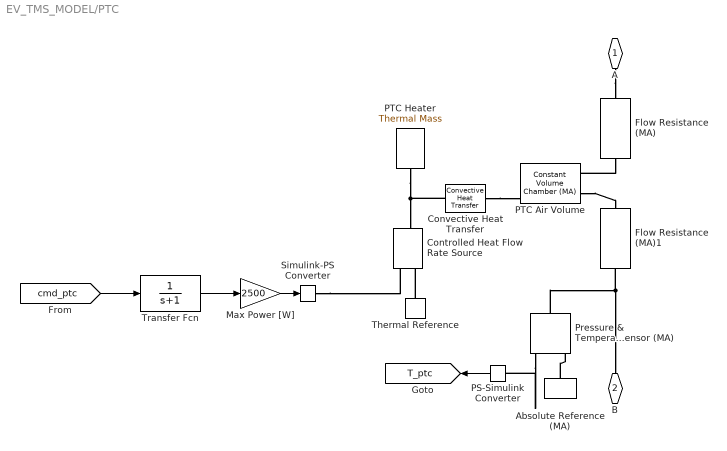
== system EV_TMS_MODEL/PTC ==
  Absolute Reference (MA) : fl_lib/Moist Air/Elements/Absolute Reference (MA)
  Controlled Heat Flow Rate Source : fl_lib/Thermal/Thermal Sources/Controlled Heat Flow Rate Source
  Convective Heat Transfer : fl_lib/Thermal/Thermal Elements/Convective Heat Transfer  thermal_type=foundation.enum.constant_variable.constant  area=1 m^2  heat_tr_coeff=200 W/(m^2 * K)  min_heat_tr_coeff=1e-3 W/(K*m^2)  T_specify=off  T_priority=None  T=0 K  T_nominal_specify=off  T_nominal_value=1  T_nominal_unit=K  Q_specify=off  Q_priority=None  Q=0 W  Q_nominal_specify=off  Q_nominal_value=1  Q_nominal_unit=W
  Flow Resistance (MA) : fl_lib/Moist Air/Elements/Flow Resistance (MA)  delta_p_nominal=2e-4 MPa  mdot_nominal=0.15 kg/s  rho_nominal=1.2 kg/m^3  area=cabin_duct_area m^2  laminar_fraction=1e-3
  Flow Resistance (MA)1 : fl_lib/Moist Air/Elements/Flow Resistance (MA)  delta_p_nominal=2e-4 MPa  mdot_nominal=0.15 kg/s  rho_nominal=1.2 kg/m^3  area=cabin_duct_area m^2  laminar_fraction=1e-3
  Max Power [W] : Gain  Gain=2500
  PS-Simulink Converter : nesl_utility/PS-Simulink Converter  PhysicalDomain=network_engine_domain  SubClassName=ps_output  LeftPortType=input  RightPortType=output  PseudoPeriodic=off  Frequencies=[]  VectorFormat=1-D array  Unit=degC  AffineConversion=on
  PTC Heater : fl_lib/Thermal/Thermal Elements/Thermal Mass  mass_type=foundation.enum.constant_variable.constant  mass=1.5 kg  sp_heat=447 J/kg/K  mass_min=1e-6 kg  num_ports=foundation.enum.numPorts2.one  m_specify=off  m_priority=High  m=1 kg  m_nominal_specify=off  m_nominal_value=1  m_nominal_unit=kg  T_specify=on  T_priority=High  T=cabin_T_init degC  T_nominal_specify=off  T_nominal_value=1  T_nominal_unit=K  Q_specify=off  Q_priority=None  Q=0 W  Q_nominal_specify=off  Q_nominal_value=1  Q_nominal_unit=W
  PTC Air Volume : fl_lib/Moist Air/Elements/Constant Volume Chamber (MA)  volume=0.001 m^3  num_ports=foundation.enum.num_ports.two  area_A=cabin_duct_area m^2  area_B=cabin_duct_area m^2  area_C=0.01 m^2  area_D=0.01 m^2  RH_ws=1  time_constant=1e-3 s  moisture_trace_gas_source=foundation.enum.moisture_trace_gas_source.none  moisture_source_spec=foundation.enum.moisture_source_spec.vapor  moisture_mass_flow=0 kg/s  moisture_temperature_spec=foundation.enum.temperature_spec.atmospheric  moisture_temperature=293.15 K  trace_gas_mass_flow=0 kg/s  trace_gas_temperature_spec=foundation.enum.temperature_spec.atmospheric  trace_gas_temperature=293.15 K  p_I_specify=on  p_I_priority=High  p_I=cabin_p_init MPa  p_I_nominal_specify=off  p_I_nominal_value=1  p_I_nominal_unit=MPa  T_I_specify=on  T_I_priority=High  T_I=cabin_T_init degC  T_I_nominal_specify=off  T_I_nominal_value=1  T_I_nominal_unit=K  RH_I_specify=on  RH_I_priority=High  RH_I=cabin_RH_init  RH_I_nominal_specify=off  RH_I_nominal_value=1  RH_I_nominal_unit=1  x_w_I_specify=off  x_w_I_priority=None  x_w_I=0  x_w_I_nominal_specify=off  x_w_I_nominal_value=1  x_w_I_nominal_unit=1  y_w_I_specify=off  y_w_I_priority=None  y_w_I=0  y_w_I_nominal_specify=off  y_w_I_nominal_value=1  y_w_I_nominal_unit=1  HR_I_specify=off  HR_I_priority=None  HR_I=0  HR_I_nominal_specify=off  HR_I_nominal_value=1  HR_I_nominal_unit=1  x_g_I_specify=on  x_g_I_priority=None  x_g_I=0  x_g_I_nominal_specify=off  x_g_I_nominal_value=1  x_g_I_nominal_unit=1  y_g_I_specify=on  y_g_I_priority=High  y_g_I=cabin_CO2_init  y_g_I_nominal_specify=off  y_g_I_nominal_value=1  y_g_I_nominal_unit=1
      settings: InternalSimscapePortConfiguration="{\"Bottom\":[],\"Left\":[{\"id\":\"A\",\"label\":\"A\",\"type\":\"foundation.moist_air.moist_air\"},{\"id\":\"B\",\"label\":\"B\",\"type\":\"foundation.moist_air.moist_air\"}],\"Right\":[{\"id\":\"W\",\"label\":\"W\",\"type\":\"output\"},{\"id\":\"F\",\"label\":\"F\",\"type\":\"output\"},{\"id\":\"H\",\"label\":\"H\",\"type\":\"foundation.thermal.thermal\"}],\"Top\":[]}"
  Pressure & Temperature Sensor (MA) : fl_lib/Moist Air/Sensors/Pressure & Temperature Sensor (MA)  reference=foundation.enum.MeasurementReference.difference  pressure=true  pressure_spec=foundation.enum.PressureMeasementSpec.Absolute  temperature=true
      settings: InternalSimscapePortConfiguration="{\"Bottom\":[{\"id\":\"T\",\"label\":\"T\",\"type\":\"output\"}],\"Left\":[{\"id\":\"A\",\"label\":\"A\",\"type\":\"foundation.moist_air.moist_air\"}],\"Right\":[{\"id\":\"B\",\"label\":\"B\",\"type\":\"foundation.moist_air.moist_air\"},{\"id\":\"P\",\"label\":\"P\",\"type\":\"output\"}],\"Top\":[]}"
  Simulink-PS Converter : nesl_utility/Simulink-PS Converter  PhysicalDomain=network_engine_domain  SubClassName=ps_input  LeftPortType=input  RightPortType=output  PseudoPeriodic=off  Frequencies=[]  NoiseDistribution=none  NoiseParameters=[]  Unit=W  AffineConversion=off  FilteringAndDerivatives=provide  SimscapeFilterOrder=1  InputFilterTimeConstant=0.001  UdotUserProvided=0
  Thermal Reference : fl_lib/Thermal/Thermal Elements/Thermal Reference
  Transfer Fcn : TransferFcn  Denominator=[1 1]
  A : PMIOPort  Side=Left
  B : PMIOPort  Port=2  Side=Right
  tag scope: T_ptc=global
  wires:
  Max Power [W]/1 -> Simulink-PS Converter/1
  Transfer Fcn/1 -> Max Power [W]/1
  [cmd_ptc] -> Transfer Fcn/1
  PS-Simulink Converter/1 -> [T_ptc]
  connections:
  PTC Heater/LConn1 -- Convective Heat Transfer/LConn1 -- Controlled Heat Flow Rate Source/LConn1
  Thermal Reference/LConn1 -- Controlled Heat Flow Rate Source/RConn2
  Pressure & Temperature Sensor (MA)/LConn1 -- Flow Resistance (MA)1/RConn1 -- B/RConn1
  Pressure & Temperature Sensor (MA)/RConn3 -- PS-Simulink Converter/LConn1
  Absolute Reference (MA)/LConn1 -- Pressure & Temperature Sensor (MA)/RConn1
  Convective Heat Transfer/RConn1 -- PTC Air Volume/RConn3
  Flow Resistance (MA)/RConn1 -- PTC Air Volume/LConn1
  PTC Air Volume/LConn2 -- Flow Resistance (MA)1/LConn1
  A/RConn1 -- Flow Resistance (MA)/LConn1
  Simulink-PS Converter/RConn1 -- Controlled Heat Flow Rate Source/RConn1

== system EV_TMS_MODEL/Refrigerant Tank ==
  Refrigerant Tank : Subsystem
      mask Display: disp(get_param(gcb, 'Name'));
  A : PMIOPort  Side=Left
  B : PMIOPort  Port=2  Side=Right
  connections:
  A/RConn1 -- Refrigerant Tank/LConn1
  Refrigerant Tank/RConn1 -- B/RConn1

== system EV_TMS_MODEL/S1 ==
  Absolute Reference (2P) : fl_lib/Two-Phase Fluid/Elements/Absolute Reference (2P)
  PS-Simulink Converter : nesl_utility/PS-Simulink Converter  PhysicalDomain=network_engine_domain  SubClassName=ps_output  LeftPortType=input  RightPortType=output  PseudoPeriodic=off  Frequencies=[]  VectorFormat=inherit  Unit=kJ/kg  AffineConversion=off
  PS-Simulink Converter1 : nesl_utility/PS-Simulink Converter  PhysicalDomain=network_engine_domain  SubClassName=ps_output  LeftPortType=input  RightPortType=output  PseudoPeriodic=off  Frequencies=[]  VectorFormat=inherit  Unit=MPa  AffineConversion=off
  Pressure & Internal Energy Sensor (2P) : fl_lib/Two-Phase Fluid/Sensors/Pressure, Temperature & Internal Energy Sensor (2P)  reference=foundation.enum.MeasurementReference.difference  pressure=true  pressure_spec=foundation.enum.PressureMeasementSpec.Absolute  temperature=false  internal_energy=true
      settings: InternalSimscapePortConfiguration="{\"Bottom\":[{\"id\":\"U\",\"label\":\"U\",\"type\":\"output\"}],\"Left\":[{\"id\":\"A\",\"label\":\"A\",\"type\":\"foundation.two_phase_fluid.two_phase_fluid\"}],\"Right\":[{\"id\":\"B\",\"label\":\"B\",\"type\":\"foundation.two_phase_fluid.two_phase_fluid\"},{\"id\":\"P\",\"label\":\"P\",\"type\":\"output\"}],\"Top\":[]}"
  Saturation Properties Sensor (2P) : fl_lib/Two-Phase Fluid/Sensors/Saturation Properties Sensor (2P)  temperature_measure=true  pressure_measure=simscape.enum.onoff.off  pressure_check=simscape.enum.assert.action.error  energy_measure=foundation.enum.EnergyMeasurement.SaturatedEnthalpy  density_measure=foundation.enum.DensityMeasurement.Off
      settings: InternalSimscapePortConfiguration="{\"Bottom\":[],\"Left\":[{\"id\":\"A\",\"label\":\"A\",\"type\":\"foundation.two_phase_fluid.two_phase_fluid\"}],\"Right\":[{\"id\":\"T_sat_liq\",\"label\":\"TL\",\"type\":\"output\"},{\"id\":\"T_sat_vap\",\"label\":\"TV\",\"type\":\"output\"}],\"Top\":[{\"id\":\"h_sat_liq\",\"label\":\"HL\",\"type\":\"output\"},{\"id\":\"h_sat_vap\",\"label\":\"HV\",\"type\":\"output\"}]}"
  Thermodynamic Properties Sensor (2P) : fl_lib/Two-Phase Fluid/Sensors/Thermodynamic Properties Sensor (2P)  temperature=true  enthalpy=true  density=false  specific_volume=true  entropy=true
      settings: InternalSimscapePortConfiguration="{\"Bottom\":[{\"id\":\"V\",\"label\":\"v\",\"type\":\"output\"},{\"id\":\"S\",\"label\":\"s\",\"type\":\"output\"}],\"Left\":[{\"id\":\"A\",\"label\":\"A\",\"type\":\"foundation.two_phase_fluid.two_phase_fluid\"}],\"Right\":[{\"id\":\"T\",\"label\":\"T\",\"type\":\"output\"},{\"id\":\"H\",\"label\":\"h\",\"type\":\"output\"}],\"Top\":[]}"
  A : PMIOPort  Side=Left
  tag scope: h1=global, p1=global
  wires:
  PS-Simulink Converter/1 -> [h1]
  PS-Simulink Converter1/1 -> [p1]
  connections:
  Pressure & Internal Energy Sensor (2P)/LConn1 -- Saturation Properties Sensor (2P)/LConn1 -- Thermodynamic Properties Sensor (2P)/LConn1 -- A/RConn1
  Absolute Reference (2P)/LConn1 -- Pressure & Internal Energy Sensor (2P)/RConn1
  PS-Simulink Converter/LConn1 -- Thermodynamic Properties Sensor (2P)/RConn2
  PS-Simulink Converter1/LConn1 -- Pressure & Internal Energy Sensor (2P)/RConn2

== system EV_TMS_MODEL/S2 ==
  Absolute Reference (2P) : fl_lib/Two-Phase Fluid/Elements/Absolute Reference (2P)
  PS-Simulink Converter : nesl_utility/PS-Simulink Converter  PhysicalDomain=network_engine_domain  SubClassName=ps_output  LeftPortType=input  RightPortType=output  PseudoPeriodic=off  Frequencies=[]  VectorFormat=inherit  Unit=kJ/kg  AffineConversion=off
  PS-Simulink Converter1 : nesl_utility/PS-Simulink Converter  PhysicalDomain=network_engine_domain  SubClassName=ps_output  LeftPortType=input  RightPortType=output  PseudoPeriodic=off  Frequencies=[]  VectorFormat=inherit  Unit=MPa  AffineConversion=off
  Pressure & Internal Energy Sensor (2P) : fl_lib/Two-Phase Fluid/Sensors/Pressure, Temperature & Internal Energy Sensor (2P)  reference=foundation.enum.MeasurementReference.difference  pressure=true  pressure_spec=foundation.enum.PressureMeasementSpec.Absolute  temperature=false  internal_energy=true
      settings: InternalSimscapePortConfiguration="{\"Bottom\":[{\"id\":\"U\",\"label\":\"U\",\"type\":\"output\"}],\"Left\":[{\"id\":\"A\",\"label\":\"A\",\"type\":\"foundation.two_phase_fluid.two_phase_fluid\"}],\"Right\":[{\"id\":\"B\",\"label\":\"B\",\"type\":\"foundation.two_phase_fluid.two_phase_fluid\"},{\"id\":\"P\",\"label\":\"P\",\"type\":\"output\"}],\"Top\":[]}"
  Saturation Properties Sensor (2P) : fl_lib/Two-Phase Fluid/Sensors/Saturation Properties Sensor (2P)  temperature_measure=true  pressure_measure=simscape.enum.onoff.off  pressure_check=simscape.enum.assert.action.error  energy_measure=foundation.enum.EnergyMeasurement.SaturatedEnthalpy  density_measure=foundation.enum.DensityMeasurement.Off
      settings: InternalSimscapePortConfiguration="{\"Bottom\":[],\"Left\":[{\"id\":\"A\",\"label\":\"A\",\"type\":\"foundation.two_phase_fluid.two_phase_fluid\"}],\"Right\":[{\"id\":\"T_sat_liq\",\"label\":\"TL\",\"type\":\"output\"},{\"id\":\"T_sat_vap\",\"label\":\"TV\",\"type\":\"output\"}],\"Top\":[{\"id\":\"h_sat_liq\",\"label\":\"HL\",\"type\":\"output\"},{\"id\":\"h_sat_vap\",\"label\":\"HV\",\"type\":\"output\"}]}"
  Thermodynamic Properties Sensor (2P) : fl_lib/Two-Phase Fluid/Sensors/Thermodynamic Properties Sensor (2P)  temperature=true  enthalpy=true  density=false  specific_volume=true  entropy=true
      settings: InternalSimscapePortConfiguration="{\"Bottom\":[{\"id\":\"V\",\"label\":\"v\",\"type\":\"output\"},{\"id\":\"S\",\"label\":\"s\",\"type\":\"output\"}],\"Left\":[{\"id\":\"A\",\"label\":\"A\",\"type\":\"foundation.two_phase_fluid.two_phase_fluid\"}],\"Right\":[{\"id\":\"T\",\"label\":\"T\",\"type\":\"output\"},{\"id\":\"H\",\"label\":\"h\",\"type\":\"output\"}],\"Top\":[]}"
  A : PMIOPort  Side=Left
  tag scope: h2=global, p2=global
  wires:
  PS-Simulink Converter/1 -> [h2]
  PS-Simulink Converter1/1 -> [p2]
  connections:
  Pressure & Internal Energy Sensor (2P)/LConn1 -- Saturation Properties Sensor (2P)/LConn1 -- Thermodynamic Properties Sensor (2P)/LConn1 -- A/RConn1
  Absolute Reference (2P)/LConn1 -- Pressure & Internal Energy Sensor (2P)/RConn1
  PS-Simulink Converter/LConn1 -- Thermodynamic Properties Sensor (2P)/RConn2
  PS-Simulink Converter1/LConn1 -- Pressure & Internal Energy Sensor (2P)/RConn2

== system EV_TMS_MODEL/S3 ==
  Absolute Reference (2P) : fl_lib/Two-Phase Fluid/Elements/Absolute Reference (2P)
  PS-Simulink Converter : nesl_utility/PS-Simulink Converter  PhysicalDomain=network_engine_domain  SubClassName=ps_output  LeftPortType=input  RightPortType=output  PseudoPeriodic=off  Frequencies=[]  VectorFormat=inherit  Unit=kJ/kg  AffineConversion=off
  PS-Simulink Converter1 : nesl_utility/PS-Simulink Converter  PhysicalDomain=network_engine_domain  SubClassName=ps_output  LeftPortType=input  RightPortType=output  PseudoPeriodic=off  Frequencies=[]  VectorFormat=inherit  Unit=MPa  AffineConversion=off
  Pressure & Internal Energy Sensor (2P) : fl_lib/Two-Phase Fluid/Sensors/Pressure, Temperature & Internal Energy Sensor (2P)  reference=foundation.enum.MeasurementReference.difference  pressure=true  pressure_spec=foundation.enum.PressureMeasementSpec.Absolute  temperature=false  internal_energy=true
      settings: InternalSimscapePortConfiguration="{\"Bottom\":[{\"id\":\"U\",\"label\":\"U\",\"type\":\"output\"}],\"Left\":[{\"id\":\"A\",\"label\":\"A\",\"type\":\"foundation.two_phase_fluid.two_phase_fluid\"}],\"Right\":[{\"id\":\"B\",\"label\":\"B\",\"type\":\"foundation.two_phase_fluid.two_phase_fluid\"},{\"id\":\"P\",\"label\":\"P\",\"type\":\"output\"}],\"Top\":[]}"
  Saturation Properties Sensor (2P) : fl_lib/Two-Phase Fluid/Sensors/Saturation Properties Sensor (2P)  temperature_measure=true  pressure_measure=simscape.enum.onoff.off  pressure_check=simscape.enum.assert.action.error  energy_measure=foundation.enum.EnergyMeasurement.SaturatedEnthalpy  density_measure=foundation.enum.DensityMeasurement.Off
      settings: InternalSimscapePortConfiguration="{\"Bottom\":[],\"Left\":[{\"id\":\"A\",\"label\":\"A\",\"type\":\"foundation.two_phase_fluid.two_phase_fluid\"}],\"Right\":[{\"id\":\"T_sat_liq\",\"label\":\"TL\",\"type\":\"output\"},{\"id\":\"T_sat_vap\",\"label\":\"TV\",\"type\":\"output\"}],\"Top\":[{\"id\":\"h_sat_liq\",\"label\":\"HL\",\"type\":\"output\"},{\"id\":\"h_sat_vap\",\"label\":\"HV\",\"type\":\"output\"}]}"
  Thermodynamic Properties Sensor (2P) : fl_lib/Two-Phase Fluid/Sensors/Thermodynamic Properties Sensor (2P)  temperature=true  enthalpy=true  density=false  specific_volume=true  entropy=true
      settings: InternalSimscapePortConfiguration="{\"Bottom\":[{\"id\":\"V\",\"label\":\"v\",\"type\":\"output\"},{\"id\":\"S\",\"label\":\"s\",\"type\":\"output\"}],\"Left\":[{\"id\":\"A\",\"label\":\"A\",\"type\":\"foundation.two_phase_fluid.two_phase_fluid\"}],\"Right\":[{\"id\":\"T\",\"label\":\"T\",\"type\":\"output\"},{\"id\":\"H\",\"label\":\"h\",\"type\":\"output\"}],\"Top\":[]}"
  A : PMIOPort  Side=Right
  tag scope: h3=global, p3=global
  wires:
  PS-Simulink Converter/1 -> [h3]
  PS-Simulink Converter1/1 -> [p3]
  connections:
  Pressure & Internal Energy Sensor (2P)/LConn1 -- Saturation Properties Sensor (2P)/LConn1 -- Thermodynamic Properties Sensor (2P)/LConn1 -- A/RConn1
  Absolute Reference (2P)/LConn1 -- Pressure & Internal Energy Sensor (2P)/RConn1
  PS-Simulink Converter/LConn1 -- Thermodynamic Properties Sensor (2P)/RConn2
  PS-Simulink Converter1/LConn1 -- Pressure & Internal Energy Sensor (2P)/RConn2
